simulink model "manning_test_merge_nonlinear"  (R2022b)
settings: Solver=VariableStepAuto  StartTime=0.0  StopTime=5*N  RelTol=1e-3
undefined symbols (not defined in the file or in its folder): yd_ds
settings Model: Creator=chuan  LastModifiedBy=chuan

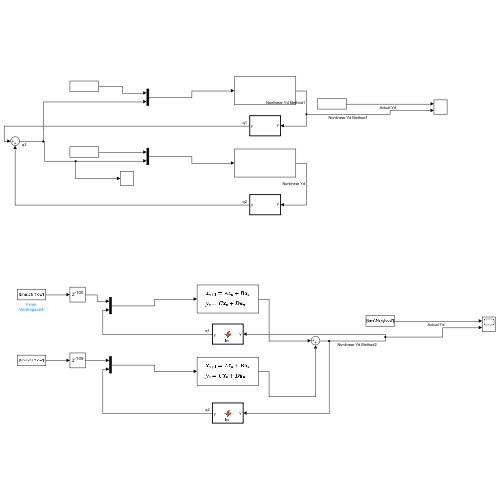
[thumbnail: Simulink's stored preview of the top-level diagram]
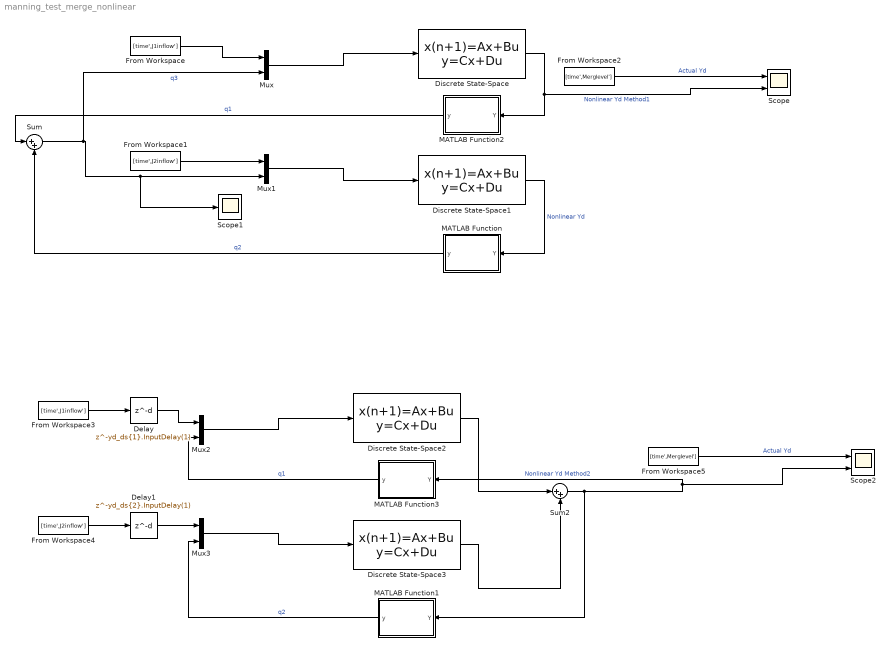
== system manning_test_merge_nonlinear ==
  Delay : Delay  DelayLength=yd_ds{1}.InputDelay(1)  InitialCondition=0
  Delay1 : Delay  DelayLength=yd_ds{2}.InputDelay(1)  InitialCondition=0
  Discrete State-Space : DiscreteStateSpace  A=yd_ds{1}.A  B=yd_ds{1}.B  C=yd_ds{1}.C  D=yd_ds{1}.D  SampleTime=yd_ds{1}.Ts
  Discrete State-Space1 : DiscreteStateSpace  A=yd_ds{2}.A  B=yd_ds{2}.B  C=yd_ds{2}.C  D=yd_ds{2}.D  SampleTime=yd_ds{2}.Ts
  Discrete State-Space2 : DiscreteStateSpace  A=yd_ds{1}.A  B=yd_ds{1}.B  C=yd_ds{1}.C  D=yd_ds{1}.D  SampleTime=yd_ds{1}.Ts
  Discrete State-Space3 : DiscreteStateSpace  A=yd_ds{2}.A  B=yd_ds{2}.B  C=yd_ds{2}.C  D=yd_ds{2}.D  SampleTime=yd_ds{2}.Ts
  From Workspace : FromWorkspace  VariableName=[time',J1inflow']
  From Workspace1 : FromWorkspace  VariableName=[time',J2inflow']
  From Workspace2 : FromWorkspace  VariableName=[time',Merglevel']
  From Workspace3 : FromWorkspace  VariableName=[time',J1inflow']
  From Workspace4 : FromWorkspace  VariableName=[time',J2inflow']
  From Workspace5 : FromWorkspace  VariableName=[time',Merglevel']
  MATLAB Function : MATLAB Function  TreatAsAtomicUnit=on
  MATLAB Function1 : MATLAB Function  TreatAsAtomicUnit=on
  MATLAB Function2 : MATLAB Function  TreatAsAtomicUnit=on
  MATLAB Function3 : MATLAB Function  TreatAsAtomicUnit=on
  Mux{,1..3} (4 alike) : Mux  Inputs=2
  Scope : Scope  NumInputPorts=2
  Scope1 : Scope
  Scope2 : Scope  NumInputPorts=2
  Sum : Sum  Inputs=|++
  Sum2 : Sum  Inputs=|++
  wires:
  Mux/1 -> Discrete State-Space/1
  From Workspace/1 -> Mux/1
  From Workspace2/1 -> Scope/1  "Actual Yd"
  From Workspace1/1 -> Mux1/1
  Mux1/1 -> Discrete State-Space1/1
  Discrete State-Space/1 -> Scope/2, MATLAB Function2/1(Y)  "Nonlinear Yd Method1"
  MATLAB Function2/1(y) -> Sum/1  "q1"
  MATLAB Function/1(y) -> Sum/2  "q2"
  Sum/1 -> Mux/2, Scope1/1, Mux1/2  "q3"
  Discrete State-Space1/1 -> MATLAB Function/1(Y)  "Nonlinear Yd"
  Discrete State-Space3/1 -> Sum2/2
  Mux3/1 -> Discrete State-Space3/1
  Discrete State-Space2/1 -> Sum2/1
  Mux2/1 -> Discrete State-Space2/1
  Sum2/1 -> MATLAB Function1/1(Y), Scope2/2, MATLAB Function3/1(Y)  "Nonlinear Yd Method2"
  From Workspace5/1 -> Scope2/1  "Actual Yd"
  MATLAB Function3/1(y) -> Mux2/2  "q1"
  MATLAB Function1/1(y) -> Mux3/2  "q2"
  From Workspace3/1 -> Delay/1
  Delay/1 -> Mux2/1
  From Workspace4/1 -> Delay1/1
  Delay1/1 -> Mux3/1

== matlab function manning_test_merge_nonlinear/MATLAB Function1 ==
  data: Y input; y output
function y = fcn(Y)
n = 0.02;
Sb = 0.0008;
B=8;
m = 1.5;

Y = max(Y,0);

y = (1/n)*(B*Y + m*Y.^2)*((B*Y + m*Y.^2)/(B + 2.*Y.*sqrt(1+m^2))).^(2/3) .* sqrt(Sb);

== matlab function manning_test_merge_nonlinear/MATLAB Function2 ==
  data: Y input; y output
function y = fcn(Y)
n = 0.02;
Sb = 0.0008;
B=8;
m = 1.5;

Y = max(Y,0);

y = (1/n)*(B*Y + m*Y.^2)*((B*Y + m*Y.^2)/(B + 2.*Y.*sqrt(1+m^2))).^(2/3) .* sqrt(Sb);

== matlab function manning_test_merge_nonlinear/MATLAB Function3 ==
  data: Y input; y output
function y = fcn(Y)
n = 0.02;
Sb = 0.0008;
B=8;
m = 1.5;

Y = max(Y,0);

y = (1/n)*(B*Y + m*Y.^2)*((B*Y + m*Y.^2)/(B + 2.*Y.*sqrt(1+m^2))).^(2/3) .* sqrt(Sb);

== matlab function manning_test_merge_nonlinear/MATLAB Function ==
  data: Y input; y output
function y = fcn(Y)
n = 0.02;
Sb = 0.0008;
B=8;
m = 1.5;

Y = max(Y,0);

y = (1/n)*(B*Y + m*Y.^2)*((B*Y + m*Y.^2)/(B + 2.*Y.*sqrt(1+m^2))).^(2/3) .* sqrt(Sb);
